simulink model "open_loop_WMR_ubuntu"  (R2024a)
settings: Solver=VariableStepAuto  StartTime=0.0  StopTime=20  RelTol=1e-3
libraries: robotlib x2
settings Model: Creator=ganes  LastModifiedBy=ganesh
settings RTWCC: GPUComputeCapability=3.5

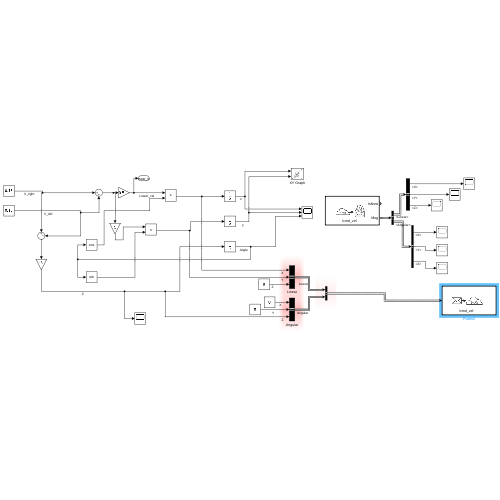
[thumbnail: Simulink's stored preview of the top-level diagram]
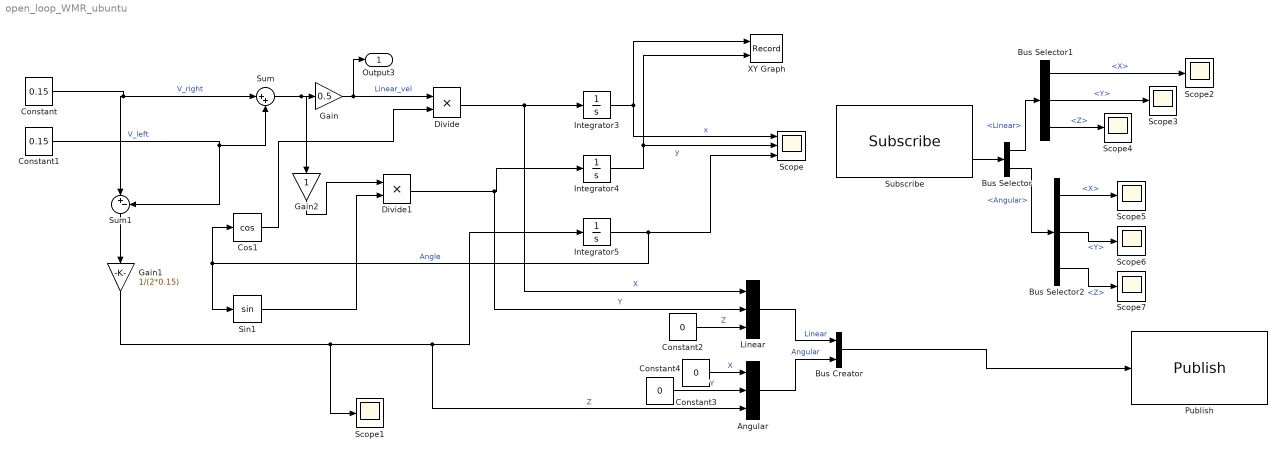
== system open_loop_WMR_ubuntu ==
  "Angular " : BusCreator  Inputs=3  OutDataTypeStr=Bus: SL_Bus_open_loop_WMR_geometry_msgs_Vector3
  Bus Creator : BusCreator  Inputs=2  OutDataTypeStr=Bus: SL_Bus_open_loop_WMR_geometry_msgs_Twist  NonVirtualBus=on
  Bus Selector : BusSelector  OutputSignals=Linear,Angular
  Bus Selector1 : BusSelector  OutputSignals=X,Y,Z
  Bus Selector2 : BusSelector  OutputSignals=X,Y,Z
  Constant : Constant  Value=0.15
  Constant1 : Constant  Value=0.15
  Constant2 : Constant  Value=0
  Constant3 : Constant  Value=0
  Constant4 : Constant  Value=0
  Cos1 : Trigonometry  Operator=cos
  Divide : Product  Inputs=**
  Divide1 : Product  Inputs=**
  Gain : Gain  Gain=0.5
  Gain1 : Gain  Gain=1/(2*0.15)
  Gain2 : Gain
  Integrator3 : Integrator
  Integrator4 : Integrator
  Integrator5 : Integrator
  Linear : BusCreator  Inputs=3  OutDataTypeStr=Bus: SL_Bus_open_loop_WMR_geometry_msgs_Vector3
  Publish : robotlib/Publish  topicSource=Select from ROS network  topic=/cmd_vel  messageType=geometry_msgs/Twist  legacyBusStruct=off  messageQueueLength=1
  Scope : Scope  NumInputPorts=3
  Scope{1..7} (7 alike) : Scope
  Sin1 : Trigonometry
  Subscribe : robotlib/Subscribe  topicSource=Select from ROS network  topic=/cmd_vel  messageType=geometry_msgs/Twist  SampleTime=-1  legacyBusStruct=off  messageQueueLength=1
  Sum : Sum  Inputs=|++
  Sum1 : Sum  Inputs=|+-
  XY Graph : Record  FileSettingsInternal="{\"entries\":[{\"content\":{\"excelSettings\":{\"content\":{},\"type\":\"Streamout.ExcelSettings\"}},\"type\":\"Streamout.FileSettingStorage\",\"uuid\":\"\"}],\"packageUris\":[\"http:\\/\\/schema.mathworks.com\\/mf0\\/streamout_blocks\\/R2020a\"],\"version\":\"1.0\"}"  Layout=[1 1]  SignalsInternal="{\"entries\":[{\"content\":{\"signals\":[{\"content\":{\"blockPath\":[],\"dimensions\":[1],\"domain\":\"\",\"lineColor\":\"#b746ff\",\"lineWidth\":2,\"port\":1,\"sid\":[\"\"],\"signalID\":1,\"signalName\":\"x\"},\"type\":\"RecordBlkView.Signal\",\"uuid\":\"\"},{\"content\":{\"blockPath\":[],\"dimensions\":[1],\"domain\":\"\",\"lineColor\":\"#64d413\",\"lineWidth\":2,\"port\":2,\"sid\":[\"\"],\"signalID\":2,\"signalName\":\"y\"},\"type\":\"RecordBlkView.Signal\",\"uuid\":\"\"}]},\"type\":\"RecordBlkView.InputSignals\",\"uuid\":\"\"}],\"packageUris\":[\"http:\\/\\/schema.mathworks.com\\/mf0\\/streamout_blocks\\/R2020a\"],\"version\":\"1.0\"}"  VisualizationBindings="{\"xyplotplugin\":{\"info\":[{\"series\":[],\"subplotID\":1}]}}"  CompatibilityTag=XY
  Output3 : Outport
  wires:
  Gain2/1 -> Divide1/1
  Sum/1 -> Gain2/1, Gain/1
  Integrator4/1 -> Scope/2, XY Graph/2  "y"
  Sum1/1 -> Gain1/1
  Constant/1 -> Sum/1, Sum1/1  "V_right"
  Sin1/1 -> Divide1/2
  Cos1/1 -> Divide/2
  Integrator3/1 -> Scope/1, XY Graph/1  "x"
  Constant1/1 -> Sum1/2, Sum/2  "V_left"
  Integrator5/1 -> Scope/3, Sin1/1, Cos1/1  "Angle"
  Gain/1 -> Output3/1, Divide/1  "Linear_vel"
  "Angular "/1 -> Bus Creator/2  "Angular"
  Linear/1 -> Bus Creator/1  "Linear"
  Bus Creator/1 -> Publish/1
  Constant4/1 -> "Angular "/2  "Y"
  Divide/1 -> Linear/1, Integrator3/1  "X"
  Divide1/1 -> Linear/2, Integrator4/1  "Y"
  Gain1/1 -> Scope1/1, "Angular "/3, Integrator5/1  "Z"
  Constant3/1 -> "Angular "/1  "X"
  Constant2/1 -> Linear/3  "Z"
  Subscribe/2 -> Bus Selector/1
  Bus Selector/1 -> Bus Selector1/1  "<Linear>"
  Bus Selector/2 -> Bus Selector2/1  "<Angular>"
  Bus Selector1/1 -> Scope2/1  "<X>"
  Bus Selector1/2 -> Scope3/1  "<Y>"
  Bus Selector1/3 -> Scope4/1  "<Z>"
  Bus Selector2/1 -> Scope5/1  "<X>"
  Bus Selector2/2 -> Scope6/1  "<Y>"
  Bus Selector2/3 -> Scope7/1  "<Z>"
